simulink model "DACModel_control101"  (R2024a)
settings: Solver=VariableStepAuto  StartTime=0.0  StopTime=Stoptime  FixedStep=0.1  RelTol=1e-3
undefined symbols (not defined in the file or in its folder): SampleTime
settings Model: Creator=sword  LastModifiedBy=Anthony Rossiter
settings RTWCC: GPUComputeCapability=3.5
settings ConfigComp: CovBoundaryAbsTol=1.0e-5

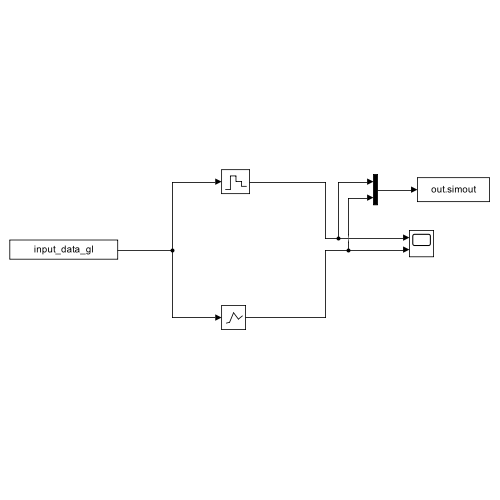
[thumbnail: Simulink's stored preview of the top-level diagram]
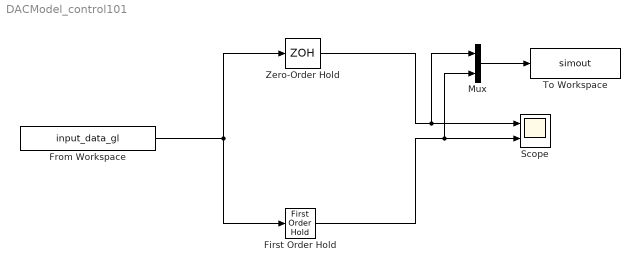
== system DACModel_control101 ==
  First Order Hold : FirstOrderHold  ErrorTolerance=inf
  From Workspace : FromWorkspace  VariableName=input_data_gl  SampleTime=SampleTime
  Mux : Mux  Inputs=2
  Scope : Scope  NumInputPorts=2
  To Workspace : ToWorkspace  VariableName=simout  SaveFormat=Structure With Time  SampleTime=SampleTime
  Zero-Order Hold : ZeroOrderHold  SampleTime=-1
  wires:
  From Workspace/1 -> First Order Hold/1, Zero-Order Hold/1
  Zero-Order Hold/1 -> Mux/1, Scope/1
  First Order Hold/1 -> Mux/2, Scope/2
  Mux/1 -> To Workspace/1
